simulink model "mpc555rt_ccp"  (Simulink 6.0)
settings: Solver=FixedStepDiscrete  StartTime=0.0  StopTime=inf  FixedStep=0.01  RelTol=1e-3
PreLoadFcn:
  | RTWConfigurationCB('preloadfcn', bdroot);mpc555rt_ccp_data
values from neighbouring files (symbols this model uses):
  STEP_PARAM = Simulink.Parameter    [mpc555rt_ccp_data.m]
libraries: mpc555toucan x1, mpc555drivers x1
CloseFcn:
  | rtwprivate ssgencode ModelCloseRequest mpc555ccpdemo
settings Model: Creator=The MathWorks Inc.  LastModifiedBy=batserve  ExtModeAutoUpdateStatusClock=off  ProdHWDeviceType=Motorola PowerPC
settings DataIOCC: SignalLoggingName=sigsOut
settings OptimizationCC: BooleanDataType=off  InlineParams=on  InlineInvariantSignals=off  OptimizeModelRefInitCode=on  LifeSpan=1
settings DebuggingCC: CheckExecutionContextPreStartOutputMsg=on  CheckExecutionContextRuntimeOutputMsg=on  SignalResolutionControl=UseLocalSettings  SolverPrmCheckMsg=none
settings HardwareCC: ProdEndianess=BigEndian  ProdHWDeviceType=Motorola PowerPC
settings ModelReferenceCC: UpdateModelReferenceTargets=IfOutOfDate
settings RTWCC: SystemTargetFile=mpc555rt.tlc  TemplateMakefile=mpc555rt.tmf  ProcessScript=mpc555rt_make_rtw_hook
settings CodeAppCC: IgnoreCustomStorageClasses=off
settings STFCustomTargetCC: TargetFcnLib=ansi_tfl_tmw.mat  GenFloatMathFcnCalls=ANSI_C  ModelReferenceCompliant=off  CombineOutputUpdateFcns=on  ERTCustomFileBanners=on  SystemTargetFile=mpc555rt.tlc
settings ERTTargetCC: TargetFcnLib=ansi_tfl_tmw.mat  GenFloatMathFcnCalls=ANSI_C  ModelReferenceCompliant=off  SupportContinuousTime=on  SupportNonInlinedSFcns=on  GenerateASAP2=on  RootIOFormat=Individual Arguments  ERTCustomFileTemplate=example_file_process.tlc  InitialValueSource=Model
settings CustomProperty: DataType=RTWOptions_EnumType__toolbox_rtw_targets_mpc555dk_mpc555dk_mpc555rt_MPC555_OPTIMIZATION_SWITCH  Value=speed
settings EnumStrPairs: String=speed

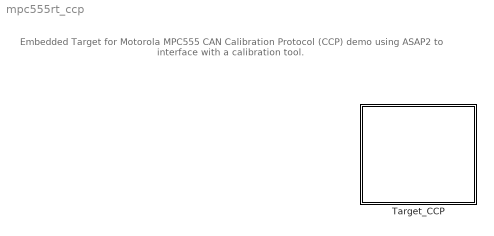
== system mpc555rt_ccp ==
  note: Embedded Target for Motorola MPC555 CAN Calibration Protocol
      | (CCP) demo using ASAP2 to interface with a calibration tool.
  Target_CCP : Subsystem  InitFcn=|  PropExecContextAcrossSSBoundary=on
      | % START RTW CONFIGURATION CODE %
      | RTWConfigurationCB('rtw_target_initfcn',gcb);
      | % END RTW CONFIGURATION CODE %
      mask Display: image(imread('target_affordance_icon.jpg'),'bottom-right')

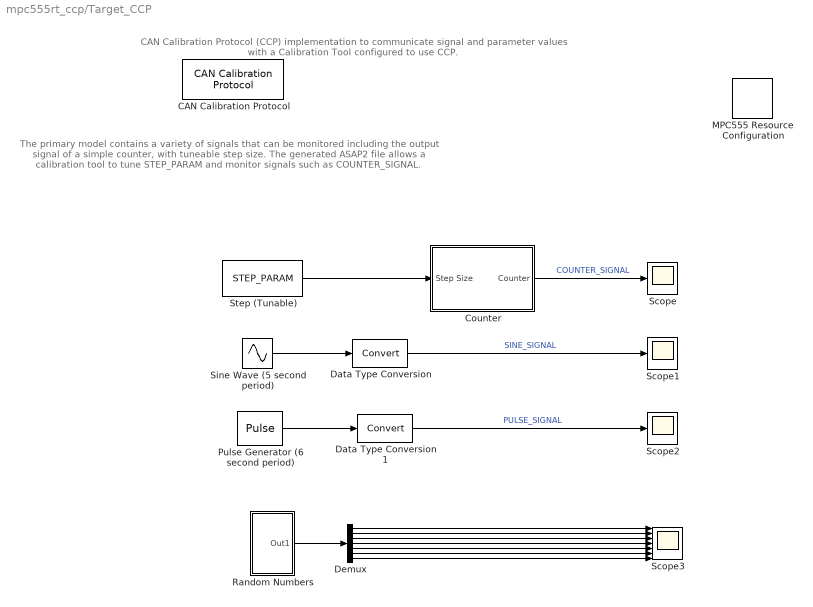
== system mpc555rt_ccp/Target_CCP ==
  note: CAN Calibration Protocol (CCP) implementation
      | to communicate signal and parameter values
      |  with a Calibration Tool configured to use CCP.
  note: The primary model contains a variety of signals that can be monitored
      | including the output signal of a simple counter, with tuneable
      | step size. The generated ASAP2 file allows a calibration tool to tune
      | STEP_PARAM and monitor signals such as COUNTER_SIGNAL.
  CAN Calibration Protocol : mpc555toucan/CAN Calibration Protocol  CCP_STATION_ID=hex2dec('1')  module=A  ccp_cro_id=hex2dec('6FA')  ccp_cro_message_type=Extended (29-bit identifier)  ccp_return_id=hex2dec('6FB')  ccp_return_message_type=Extended (29-bit identifier)  TOTAL_NUM_ODTS=8  cro_sample_time=0.01
  Counter : Subsystem  PropExecContextAcrossSSBoundary=on
  Data Type Conversion : DataTypeConversion  OutDataTypeMode=int8  SaturateOnIntegerOverflow=on  RndMeth=Zero
  Data Type Conversion1 : DataTypeConversion  OutDataTypeMode=uint16  SaturateOnIntegerOverflow=on  RndMeth=Zero
  Demux : Demux  Outputs=7
  MPC555 Resource Configuration : mpc555drivers/MPC555 Resource Configuration  Tag=RTW CONFIGURATION BLOCK  Priority=-100000  oldParentName=mpc555rt_ccp/Target_CCP  oldBlockName=|  defaultConfigLibrary=mpc555drivers
      | mpc555rt_ccp/Target_CCP/MPC555
      | Resource
      | Configuration
  Pulse Generator (6 second period) : DiscretePulseGenerator  Amplitude=60000  Period=12  PulseWidth=4  SampleTime=0.5
  Random Numbers : Subsystem  PropExecContextAcrossSSBoundary=on
  Scope : Scope
      settings: YMin=-130  YMax=0
  Scope1 : Scope
      settings: YMin=-130  YMax=0
  Scope2 : Scope
      settings: YMin=-130  YMax=0  SaveName=ScopeData2
  Scope3 : Scope  NumInputPorts=7
      settings: YMin=-130~-5~-5~-5~-5~-5~-5  YMax=0~5~5~5~5~5~5  SaveName=ScopeData3
  Sine Wave (5 second period) : Sin  SineType=Sample based  Amplitude=125  Samples=50  SampleTime=0.1
  Step (Tunable) : Constant  Value=STEP_PARAM
  wires:
  Step (Tunable)/1 -> Counter/1(Step Size)
  Counter/1(Counter) -> Scope/1  "COUNTER_SIGNAL"
  Sine Wave (5 second period)/1 -> Data Type Conversion/1
  Data Type Conversion/1 -> Scope1/1  "SINE_SIGNAL"
  Pulse Generator (6 second period)/1 -> Data Type Conversion1/1
  Data Type Conversion1/1 -> Scope2/1  "PULSE_SIGNAL"
  Random Numbers/1(Out1) -> Demux/1
  Demux/1 -> Scope3/1
  Demux/2 -> Scope3/2
  Demux/3 -> Scope3/3
  Demux/4 -> Scope3/4
  Demux/5 -> Scope3/5
  Demux/6 -> Scope3/6
  Demux/7 -> Scope3/7

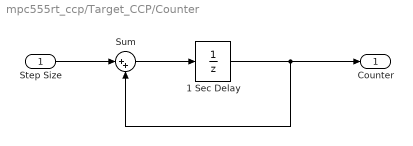
== system mpc555rt_ccp/Target_CCP/Counter ==
  Step Size : Inport  Port=1  LatchInput=off
  1 Sec Delay : UnitDelay
  Sum : Sum  Inputs=|++  SaturateOnIntegerOverflow=on  InputSameDT=on
  Counter : Outport
  wires:
  Sum/1 -> 1 Sec Delay/1
  1 Sec Delay/1 -> Sum/2, Counter/1
  Step Size/1 -> Sum/1

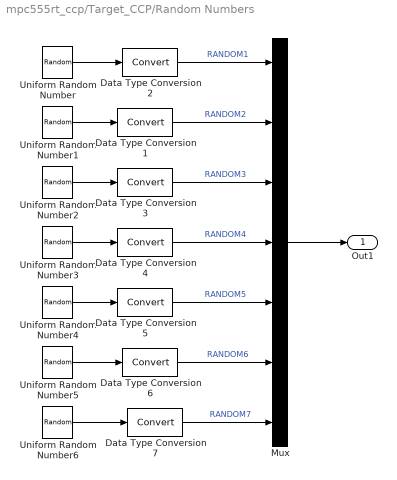
== system mpc555rt_ccp/Target_CCP/Random Numbers ==
  Data Type Conversion{1..7} (7 alike) : DataTypeConversion  OutDataTypeMode=uint8  SaturateOnIntegerOverflow=on  RndMeth=Zero
  Mux : Mux  Inputs=7
  Uniform Random Number : UniformRandomNumber  Minimum=0  Maximum=10  Seed=[0]  SampleTime=1
  Uniform Random Number1 : UniformRandomNumber  Minimum=0  Maximum=10  Seed=[1]  SampleTime=1
  Uniform Random Number2 : UniformRandomNumber  Minimum=0  Maximum=10  Seed=[2]  SampleTime=1
  Uniform Random Number3 : UniformRandomNumber  Minimum=0  Maximum=10  Seed=[3]  SampleTime=1
  Uniform Random Number4 : UniformRandomNumber  Minimum=0  Maximum=10  Seed=[4]  SampleTime=1
  Uniform Random Number5 : UniformRandomNumber  Minimum=0  Maximum=10  Seed=[5]  SampleTime=1
  Uniform Random Number6 : UniformRandomNumber  Minimum=0  Maximum=10  Seed=[6]  SampleTime=1
  Out1 : Outport
  wires:
  Uniform Random Number/1 -> Data Type Conversion2/1
  Data Type Conversion2/1 -> Mux/1  "RANDOM1"
  Data Type Conversion1/1 -> Mux/2  "RANDOM2"
  Data Type Conversion3/1 -> Mux/3  "RANDOM3"
  Data Type Conversion4/1 -> Mux/4  "RANDOM4"
  Data Type Conversion5/1 -> Mux/5  "RANDOM5"
  Data Type Conversion6/1 -> Mux/6  "RANDOM6"
  Data Type Conversion7/1 -> Mux/7  "RANDOM7"
  Uniform Random Number1/1 -> Data Type Conversion1/1
  Uniform Random Number2/1 -> Data Type Conversion3/1
  Uniform Random Number3/1 -> Data Type Conversion4/1
  Uniform Random Number4/1 -> Data Type Conversion5/1
  Uniform Random Number5/1 -> Data Type Conversion6/1
  Uniform Random Number6/1 -> Data Type Conversion7/1
  Mux/1 -> Out1/1
